simulink model "IPMSM_FOC_r2020b"  (R2020b)
settings: Solver=FixedStepDiscrete  StartTime=0.0  StopTime=20  FixedStep=Ts  RelTol=1e-3  EnableMultiTasking=on
InitFcn:
  | Ts=50e-6;     %simulation time step
  | kp = 1e-4;   %proportional gain
  | ki =0.01e-1;     %integral gain
  | fsw = 1e3;     %switching frequency
undefined symbols (not defined in the file): DiscIntNeverNeededParam
libraries: powerlib x7, powerlib_meascontrol x6
Description:
  | Copyright 2008-2019 The MathWorks, Inc.
settings Model: SimulationMode=external  ExtModeEnableFloating=off  Creator=MathWorks  LastModifiedBy=Research
settings SolverCC: ConcurrentTasks=on  PositivePriorityOrder=on  AutoInsertRateTranBlk=on
settings DataIOCC: LimitDataPoints=on  SaveFormat=Array  SignalLoggingSaveFormat=ModelDataLogs  SaveOutput=off  SignalLogging=off  SaveTime=off  ReturnWorkspaceOutputs=off  SignalLoggingName=sigsOut
settings OptimizationCC: BlockReduction=off  OptimizeBlockIOStorage=off  ExpressionDepthLimit=2147483647  InitFltsAndDblsToZero=on
settings DebuggingCC: UnderspecifiedInitializationDetection=Classic  MergeDetectMultiDrivingBlocksExec=none  CheckExecutionContextPreStartOutputMsg=on  SignalResolutionControl=TryResolveAllWithWarning  TasksWithSamePriorityMsg=none  FcnCallInpInsideContextMsg=warning  AllowSymbolicDim=off  StateNameClashWarn=warning  SFUnexpectedBacktrackingDiag=warning  SFNoUnconditionalDefaultTransitionDiag=warning  SFExecutionAtInitializationDiag=none  ArithmeticOperatorsInVariantConditions=warning
settings HardwareCC: ProdBitPerLong=64  ProdLongLongMode=on  ProdHWDeviceType=Intel->x86-64 (Linux 64)  TargetBitPerPointer=64  TargetBitPerSizeT=64  TargetBitPerPtrDiffT=64  TargetLongLongMode=on  TargetIntDivRoundTo=Zero  TargetEndianess=LittleEndian  TargetWordSize=64  TargetHWDeviceType=MATLAB Host
settings ModelReferenceCC: PropagateSignalLabelsOutOfModel=off
settings SFSimCC: SimUseLocalCustomCode=off  CustomCodeUndefinedFunction=UseInterfaceOnly
settings RTWCC: Description=Simulink Real-Time  SystemTargetFile=slrealtime.tlc  TemplateMakefile=slrealtime_default_tmf  RTWUseLocalCustomCode=off  Toolchain=Simulink Real-Time Toolchain  BuildConfiguration=Faster Runs  CodeExecutionProfiling=on  TargetLang=C++
settings CodeAppCC: StateflowObjectComments=on
settings ConfigComp: CovMetricSettings=dw  CovSaveCumulativeToWorkspaceVar=on  CovSaveSingleToWorkspaceVar=on  CovExternalEMLEnable=off  CovSFcnEnable=off
settings SimscapeCC: SimscapeNormalizeSystem=off

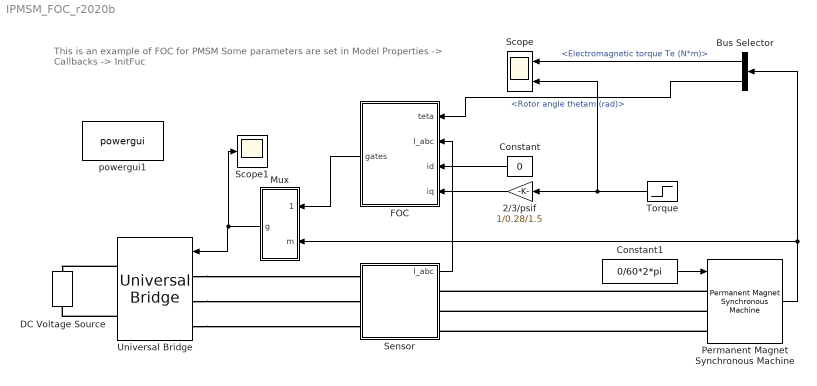
== system IPMSM_FOC_r2020b ==
  note: This is an example of FOC for PMSM
      | Some parameters are set in Model Properties -> Callbacks -> InitFuc
  2/3/psif : Gain  Gain=1/0.28/1.5  SaturateOnIntegerOverflow=on  OutDataTypeStr=Inherit: Same as input  ParamDataTypeStr=Inherit: Same as input
  Bus Selector : BusSelector  OutputSignals=Electromagnetic torque Te (N*m),Rotor angle thetam (rad)
  Constant : Constant  Value=0
  Constant1 : Constant  Value=0/60*2*pi
  DC Voltage Source : powerlib/Electrical Sources/DC Voltage Source  Amplitude=400  Measurements=None
  FOC : Subsystem
  Mux : Subsystem
  Permanent Magnet Synchronous Machine : powerlib/Machines/Permanent Magnet Synchronous Machine  NbPhases=3  FluxDistribution=Sinusoidal  RotorType=Salient-pole  MechanicalLoad=Speed w  PresetModel=No  ShowDetailedParameters=on  MeasurementBus=off  Resistance=0.1  Inductance=8.5e-3  dqInductances="[0.00006  0.00008]*10"  La=0.000395  MachineConstant=Flux linkage established by magnets (V.s)  Flux=0.28  VoltageCst=50.7864  TorqueCst=0.42  Flat=120  Mechanical=[0.0027 0.0004924 1 0]  PolePairs=1  InitialConditions=[0,0, 0,0]  InitialConditions5ph=[0 0 0 0 0 0]  RefAngle=90 degrees behind phase A axis (modified Park)  IterativeDiscreteModel=Trapezoidal non iterative  TsBlock=-1  TsPowergui=0
  Scope : Scope  NumInputPorts=2
  Scope1 : Scope
  Sensor : Subsystem
  Torque : Step  Time=0.3  After=300
  Universal Bridge : powerlib/Power Electronics/Universal Bridge  Arms=3  SnubberResistance=5000  SnubberCapacitance=inf  Device=Ideal Switches  Ron=1e-4  Lon=0  ForwardVoltages="[  0  0  ]"  ForwardVoltage=0  GTOparameters=[ 10e-6 , 20e-6 ]  IGBTparameters=[ 1e-6 , 2e-6 ]  Measurements=None  Measurements_2=None  converterType=Rectifier
  powergui1 : powerlib/powergui  Priority=1  SimulationMode=Discrete  SampleTime=Ts  frequency=60  Iterations=50  frequencyindice=0  Pbase=100e6  ErrMax=1e-4  UnitsV=kV  UnitsW=MW  buscounter=0  FunctionMessages=off  echomessages=off  EnableUseOfTLC=off  CurrentSourceSwitches=off  DisableSnubberDevices=off  DisableRonSwitches=off  DisableVfSwitches=off  DisplayEquations=off  AutomaticDiscreteSolvers=off  SolverType=Tustin  Interpol=off  ExternalGateDelay=off  methode=off  Ts=100  x0status=blocks  SPID=on  SwTol=0  HookPort=off  NonlinearTolerance=1e-4  nMaxIteration=100  ContinueOnMaxIteration=off  RestoreLinks=warning  ResistiveCurrentMeasurement=off  Frange=[0:2:500]  Ylog=off  Xlog=on  ShowGrid=off  save=off  variable=ZData  structure=0  ZoomFFT=off  StartTime=0.0  cycles=1  DisplayStyle=1  fundamental=60  FreqAxis=off  MaxFrequency=1000  frequencyindicesteady=1  RmsSteady=1  display=off
  wires:
  Bus Selector/2 -> FOC/1(teta)  "<Rotor angle thetam (rad)>"
  Permanent Magnet Synchronous Machine/1 -> Bus Selector/1, Mux/2(m)
  FOC/1(gates) -> Mux/1(gates)
  Sensor/1(I_abc) -> FOC/2(I_abc)
  Constant1/1 -> Permanent Magnet Synchronous Machine/1
  Constant/1 -> FOC/3(id)
  Mux/1(g) -> Scope1/1, Universal Bridge/1
  2/3/psif/1 -> FOC/4(iq)
  Bus Selector/1 -> Scope/1  "<Electromagnetic torque Te (N*m)>"
  Torque/1 -> 2/3/psif/1, Scope/2
  connections:
  Universal Bridge/RConn2 -- DC Voltage Source/LConn1
  Universal Bridge/LConn3 -- Sensor/LConn3
  Universal Bridge/LConn1 -- Sensor/LConn1
  Universal Bridge/LConn2 -- Sensor/LConn2
  Permanent Magnet Synchronous Machine/LConn1 -- Sensor/RConn1
  Permanent Magnet Synchronous Machine/LConn2 -- Sensor/RConn2
  Permanent Magnet Synchronous Machine/LConn3 -- Sensor/RConn3
  Universal Bridge/RConn1 -- DC Voltage Source/RConn1

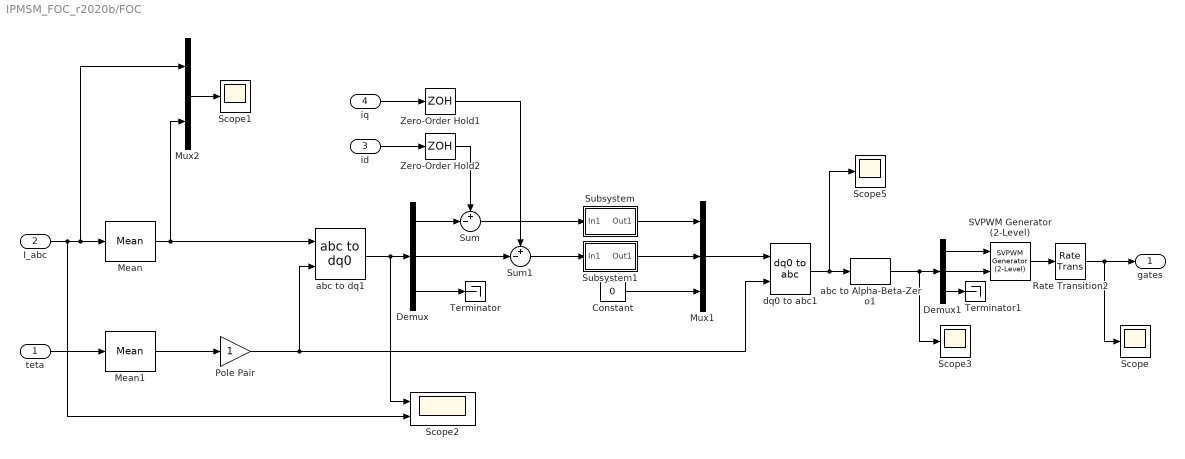
== system IPMSM_FOC_r2020b/FOC ==
  teta : Inport
  I_abc : Inport  Port=2
  id : Inport  Port=3
  iq : Inport  Port=4
  Constant : Constant  Value=0
  Demux : Demux  Outputs=3
  Demux1 : Demux  Outputs=3
  Mean : powerlib_meascontrol/Measurements/Mean  Freq=fsw  Vinit=0  Ts=Ts
  Mean1 : powerlib_meascontrol/Measurements/Mean  Freq=fsw  Vinit=0  Ts=Ts
  Mux1 : Mux  Inputs=[1 1 1]
  Mux2 : Mux  Inputs=2
  Pole Pair : Gain  SaturateOnIntegerOverflow=on  OutDataTypeStr=Inherit: Same as input  ParamDataTypeStr=Inherit: Same as input
  Rate Transition2 : RateTransition
  SVPWM Generator (2-Level) : powerlib_meascontrol/Pulse & Signal Generators/SVPWM Generator (2-Level)  InputType=alpha-beta components  SwitchingPattern=Pattern #2  Fc=fsw  ParUref=[0.8 -30 50]  Ts=Ts
      settings: SourceProductBaseCode=PS
  Scope{,1,3,5} (4 alike) : Scope
  Scope2 : Scope  NumInputPorts=2
  Subsystem : Subsystem
  Subsystem1 : Subsystem
  Sum : Sum  Inputs=+-|
  Sum1 : Sum  Inputs=+-|
  Terminator : Terminator
  Terminator1 : Terminator
  Zero-Order Hold1 : ZeroOrderHold  SampleTime=1/fsw
  Zero-Order Hold2 : ZeroOrderHold  SampleTime=1/fsw
  abc to Alpha-Beta-Zero1 : powerlib_meascontrol/Transformations/abc to Alpha-Beta-Zero
  abc to dq1 : powerlib_meascontrol/Transformations/abc to dq0  Alignment=90 degrees behind phase A axis
  dq0 to abc1 : powerlib_meascontrol/Transformations/dq0 to abc  Alignment=Aligned with phase A axis
  gates : Outport  VectorParamsAs1DForOutWhenUnconnected=off
  wires:
  abc to dq1/1 -> Demux/1, Scope2/1
  Demux/2 -> Sum1/2
  dq0 to abc1/1 -> Scope5/1, abc to Alpha-Beta-Zero1/1
  abc to Alpha-Beta-Zero1/1 -> Demux1/1, Scope3/1
  Mean1/1 -> Pole Pair/1
  Pole Pair/1 -> dq0 to abc1/2, abc to dq1/2
  Demux1/1 -> SVPWM Generator (2-Level)/1
  Mean/1 -> abc to dq1/1, Mux2/2
  SVPWM Generator (2-Level)/1 -> Rate Transition2/1
  Demux/3 -> Terminator/1
  iq/1 -> Zero-Order Hold1/1
  Rate Transition2/1 -> gates/1, Scope/1
  id/1 -> Zero-Order Hold2/1
  Demux1/2 -> SVPWM Generator (2-Level)/2
  Subsystem/1(Out1) -> Mux1/1
  Subsystem1/1(Out1) -> Mux1/2
  Constant/1 -> Mux1/3
  teta/1 -> Mean1/1
  Sum1/1 -> Subsystem1/1(In1)
  I_abc/1 -> Scope2/2, Mean/1, Mux2/1
  Demux/1 -> Sum/2
  Sum/1 -> Subsystem/1(In1)
  Demux1/3 -> Terminator1/1
  Zero-Order Hold1/1 -> Sum1/1
  Zero-Order Hold2/1 -> Sum/1
  Mux2/1 -> Scope1/1
  Mux1/1 -> dq0 to abc1/1

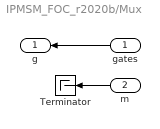
== system IPMSM_FOC_r2020b/Mux ==
  gates : Inport
  m : Inport  Port=2
  Terminator : Terminator
  g : Outport  VectorParamsAs1DForOutWhenUnconnected=off
  wires:
  m/1 -> Terminator/1
  gates/1 -> g/1

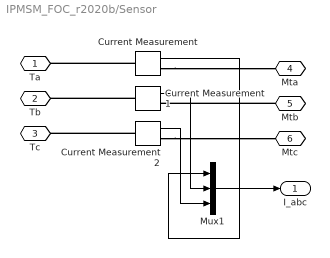
== system IPMSM_FOC_r2020b/Sensor ==
  Current Measurement : powerlib/Measurements/Current Measurement  PhasorSimulation=off  OutputType=Complex  PSBequivalent=0
  Current Measurement1 : powerlib/Measurements/Current Measurement  PhasorSimulation=off  OutputType=Complex  PSBequivalent=0
  Current Measurement2 : powerlib/Measurements/Current Measurement  PhasorSimulation=off  OutputType=Complex  PSBequivalent=0
  Mux1 : Mux  Inputs=3
  Ta : PMIOPort  Side=Left
  Tb : PMIOPort  Port=2  Side=Left
  Tc : PMIOPort  Port=3  Side=Left
  Mta : PMIOPort  Port=4  Side=Right
  Mtb : PMIOPort  Port=5  Side=Right
  Mtc : PMIOPort  Port=6  Side=Right
  I_abc : Outport  VectorParamsAs1DForOutWhenUnconnected=off
  wires:
  Current Measurement1/1 -> Mux1/2
  Current Measurement/1 -> Mux1/1
  Current Measurement2/1 -> Mux1/3
  Mux1/1 -> I_abc/1
  connections:
  Mtb/RConn1 -- Current Measurement1/RConn1
  Current Measurement1/LConn1 -- Tb/RConn1
  Current Measurement/RConn1 -- Mta/RConn1
  Current Measurement/LConn1 -- Ta/RConn1
  Current Measurement2/LConn1 -- Tc/RConn1
  Current Measurement2/RConn1 -- Mtc/RConn1

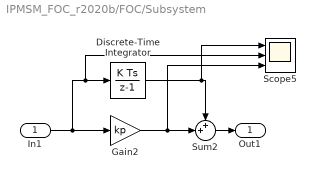
== system IPMSM_FOC_r2020b/FOC/Subsystem ==
  In1 : Inport
  Discrete-Time Integrator : DiscreteIntegrator  gainval=ki  SampleTime=-1  LimitOutput=on  UpperSaturationLimit=1  LowerSaturationLimit=-1  ICPrevOutput=DiscIntNeverNeededParam  ICPrevScaledInput=DiscIntNeverNeededParam
  Gain2 : Gain  Gain=kp  SaturateOnIntegerOverflow=on  OutDataTypeStr=Inherit: Same as input  ParamDataTypeStr=Inherit: Same as input
  Scope5 : Scope  NumInputPorts=3
  Sum2 : Sum  Inputs=++|
  Out1 : Outport  VectorParamsAs1DForOutWhenUnconnected=off
  wires:
  Gain2/1 -> Scope5/3, Sum2/2
  In1/1 -> Scope5/2, Discrete-Time Integrator/1, Gain2/1
  Sum2/1 -> Out1/1
  Discrete-Time Integrator/1 -> Scope5/1, Sum2/1

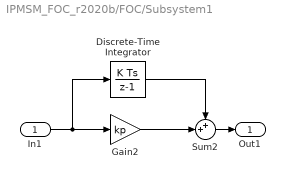
== system IPMSM_FOC_r2020b/FOC/Subsystem1 ==
  In1 : Inport
  Discrete-Time Integrator : DiscreteIntegrator  gainval=ki  SampleTime=-1  LimitOutput=on  UpperSaturationLimit=1  LowerSaturationLimit=-1  ICPrevOutput=DiscIntNeverNeededParam  ICPrevScaledInput=DiscIntNeverNeededParam
  Gain2 : Gain  Gain=kp  SaturateOnIntegerOverflow=on  OutDataTypeStr=Inherit: Same as input  ParamDataTypeStr=Inherit: Same as input
  Sum2 : Sum  Inputs=++|
  Out1 : Outport  VectorParamsAs1DForOutWhenUnconnected=off
  wires:
  Gain2/1 -> Sum2/2
  In1/1 -> Discrete-Time Integrator/1, Gain2/1
  Sum2/1 -> Out1/1
  Discrete-Time Integrator/1 -> Sum2/1
